simulink model "Project_Simulation_2"  (R2020a)
settings: Solver=ode45  StartTime=0.0  StopTime=1  RelTol=1e-3
libraries: powerlib x20
settings Model: Creator=Kryptic  LastModifiedBy=Kryptic

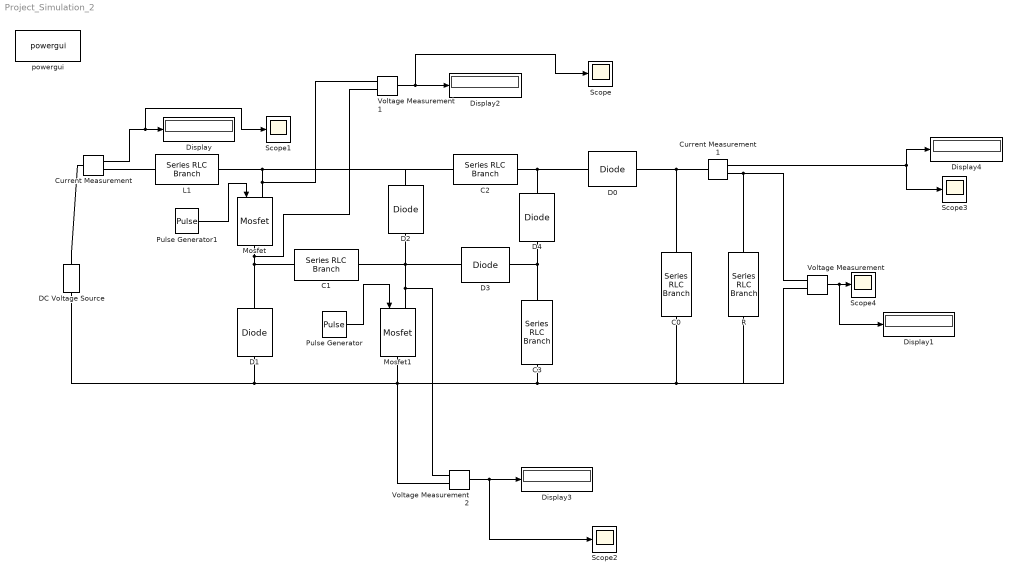
== system Project_Simulation_2 ==
  C0 : powerlib/Elements/Series RLC Branch  LConnTagsString=__new0  RConnTagsString=__new0  BranchType=C  Resistance=1  Inductance=1e-3  SetiL0=off  InitialCurrent=0  Capacitance=6.23e-7  Setx0=off  InitialVoltage=0  Measurements=None
  C1 : powerlib/Elements/Series RLC Branch  LConnTagsString=__new0  RConnTagsString=__new0  BranchType=C  Resistance=1  Inductance=1e-3  SetiL0=off  InitialCurrent=0  Capacitance=3.96e-6  Setx0=off  InitialVoltage=0  Measurements=None
  C2 : powerlib/Elements/Series RLC Branch  LConnTagsString=__new0  RConnTagsString=__new0  BranchType=C  Resistance=1  Inductance=1e-3  SetiL0=off  InitialCurrent=0  Capacitance=2.2e-7  Setx0=off  InitialVoltage=0  Measurements=None
  C3 : powerlib/Elements/Series RLC Branch  LConnTagsString=__new0  RConnTagsString=__new0  BranchType=C  Resistance=1  Inductance=1e-3  SetiL0=off  InitialCurrent=0  Capacitance=4.4e-7  Setx0=off  InitialVoltage=0  Measurements=None
  Current Measurement : powerlib/Measurements/Current Measurement  PhasorSimulation=off  OutputType=Complex  PSBequivalent=0
  Current Measurement1 : powerlib/Measurements/Current Measurement  PhasorSimulation=off  OutputType=Complex  PSBequivalent=0
  D0 : powerlib/Power Electronics/Diode  Ron=0.001  Lon=0  Vf=1.50  IC=0  UseSnubber=0  Rs=500  Cs=250e-9  Measurements=off
  D1 : powerlib/Power Electronics/Diode  Ron=0.001  Lon=0  Vf=0.86  IC=0  UseSnubber=0  Rs=500  Cs=250e-9  Measurements=off
  D2 : powerlib/Power Electronics/Diode  Ron=0.001  Lon=0  Vf=0.86  IC=0  UseSnubber=0  Rs=500  Cs=250e-9  Measurements=off
  D3 : powerlib/Power Electronics/Diode  Ron=0.001  Lon=0  Vf=0.86  IC=0  UseSnubber=0  Rs=500  Cs=250e-9  Measurements=off
  D4 : powerlib/Power Electronics/Diode  Ron=0.001  Lon=0  Vf=1.50  IC=0  UseSnubber=0  Rs=500  Cs=250e-9  Measurements=off
  DC Voltage Source : powerlib/Electrical Sources/DC Voltage Source  Amplitude=12  Measurements=None
  Display{,1..4} (5 alike) : Display
  L1 : powerlib/Elements/Series RLC Branch  LConnTagsString=__new0  RConnTagsString=__new0  BranchType=L  Resistance=1  Inductance=5.6e-3  SetiL0=off  InitialCurrent=0  Capacitance=1e-6  Setx0=off  InitialVoltage=0  Measurements=None
  Mosfet : powerlib/Power Electronics/Mosfet  Ron=8e-3  Lon=0  Rd=0.01  Vfd=0  IC=0  Rs=1e5  Cs=inf  Measurements=off
  Mosfet1 : powerlib/Power Electronics/Mosfet  Ron=8e-3  Lon=0  Rd=0.01  Vfd=0  IC=0  Rs=1e5  Cs=inf  Measurements=off
  Pulse Generator : DiscretePulseGenerator  PulseType=Time based  Period=1/25000  PulseWidth=42.1
  Pulse Generator1 : DiscretePulseGenerator  PulseType=Time based  Period=1/25000  PulseWidth=42.1
  R : powerlib/Elements/Series RLC Branch  LConnTagsString=__new0  RConnTagsString=__new0  BranchType=R  Resistance=2700  Inductance=1e-3  SetiL0=off  InitialCurrent=0  Capacitance=1e-6  Setx0=off  InitialVoltage=0  Measurements=None
  Scope{,1..4} (5 alike) : Scope
  Voltage Measurement : powerlib/Measurements/Voltage Measurement  PhasorSimulation=off  OutputType=Complex  PSBequivalent=0
  Voltage Measurement1 : powerlib/Measurements/Voltage Measurement  PhasorSimulation=off  OutputType=Complex  PSBequivalent=0
  Voltage Measurement2 : powerlib/Measurements/Voltage Measurement  PhasorSimulation=off  OutputType=Complex  PSBequivalent=0
  powergui : powerlib/powergui  Priority=1  SimulationMode=Discrete  SampleTime=1e-6  frequency=60  Iterations=50  frequencyindice=0  Pbase=100e6  ErrMax=1e-4  UnitsV=kV  UnitsW=MW  buscounter=0  FunctionMessages=off  echomessages=off  EnableUseOfTLC=off  CurrentSourceSwitches=off  DisableSnubberDevices=off  DisableRonSwitches=off  DisableVfSwitches=off  DisplayEquations=off  AutomaticDiscreteSolvers=off  SolverType=Tustin/Backward Euler (TBE)  Interpol=off  ExternalGateDelay=off  methode=off  Ts=100  x0status=blocks  SPID=on  SwTol=0  HookPort=off  NonlinearTolerance=1e-4  nMaxIteration=100  ContinueOnMaxIteration=off  RestoreLinks=warning  ResistiveCurrentMeasurement=off  Frange=[0:2:500]  Ylog=off  Xlog=on  ShowGrid=off  save=off  variable=ZData  structure=0  ZoomFFT=off  StartTime=0.0  cycles=1  DisplayStyle=1  fundamental=60  FreqAxis=off  MaxFrequency=1000  frequencyindicesteady=1  RmsSteady=1  display=off
  wires:
  Pulse Generator1/1 -> Mosfet/1
  Current Measurement/1 -> Scope1/1, Display/1
  Voltage Measurement/1 -> Display1/1, Scope4/1
  Pulse Generator/1 -> Mosfet1/1
  Voltage Measurement1/1 -> Scope/1, Display2/1
  Voltage Measurement2/1 -> Scope2/1, Display3/1
  Current Measurement1/1 -> Display4/1, Scope3/1
  connections:
  Voltage Measurement2/LConn2 -- C0/RConn1 -- R/RConn1 -- Voltage Measurement/LConn2 -- C3/RConn1 -- Mosfet1/RConn1 -- DC Voltage Source/LConn1 -- D1/RConn1
  Mosfet/LConn1 -- C2/LConn1 -- D2/LConn1 -- L1/RConn1 -- Voltage Measurement1/LConn1
  D1/LConn1 -- C1/LConn1 -- Voltage Measurement1/LConn2 -- Mosfet/RConn1
  Mosfet1/LConn1 -- Voltage Measurement2/LConn1 -- C1/RConn1 -- D2/RConn1 -- D3/LConn1
  D0/LConn1 -- C2/RConn1 -- D4/RConn1
  D3/RConn1 -- D4/LConn1 -- C3/LConn1
  C0/LConn1 -- D0/RConn1 -- Current Measurement1/LConn1
  Current Measurement/RConn1 -- L1/LConn1
  DC Voltage Source/RConn1 -- Current Measurement/LConn1
  Voltage Measurement/LConn1 -- Current Measurement1/RConn1 -- R/LConn1
